simulink model "Diagrama_de_Blocos_2"  (R2018b)
settings: Solver=FixedStepAuto  StartTime=0.0  StopTime=300  FixedStep=1e-3  RelTol=1e-3
undefined symbols (not defined in the file): A, du1, hb, k1, k2, u1b, u2
settings Model: Creator=davi2  LastModifiedBy=davi2
settings DataIOCC: SaveOutput=off  SignalLogging=off  DSMLogging=off  TimeSaveName=t

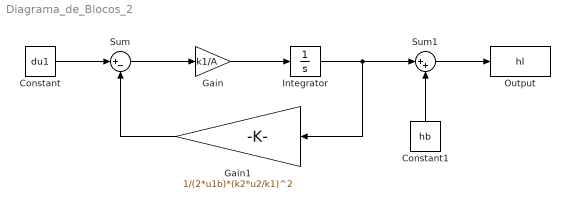
== system Diagrama_de_Blocos_2 ==
  Constant : Constant  Value=du1
  Constant1 : Constant  Value=hb
  Gain : Gain  Gain=k1/A
  Gain1 : Gain  Gain=1/(2*u1b)*(k2*u2/k1)^2
  Integrator : Integrator
  Output : ToWorkspace  VariableName=hl  SampleTime=-1
  Sum : Sum  Inputs=|+-
  Sum1 : Sum  Inputs=|++
  wires:
  Sum/1 -> Gain/1
  Gain/1 -> Integrator/1
  Integrator/1 -> Sum1/1, Gain1/1
  Gain1/1 -> Sum/2
  Sum1/1 -> Output/1
  Constant/1 -> Sum/1
  Constant1/1 -> Sum1/2
